simulink model "digital_example_R2017b"  (R2017b)
settings: Solver=VariableStepAuto  StartTime=0.0  StopTime=2  MaxStep=0.001  RelTol=1e-3
undefined symbols (not defined in the file): Kp, T0
settings Model: Creator=Anton Mayorov  LastModifiedBy=bedla

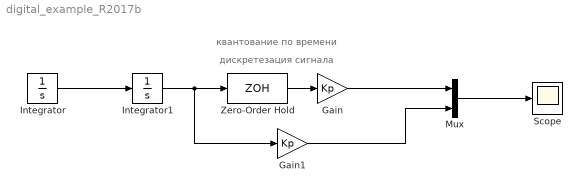
== system digital_example_R2017b ==
  note: дискретезация сигнала
  note: квантование по времени
  Gain : Gain  Gain=Kp
  Gain1 : Gain  Gain=Kp
  Integrator : Integrator  InitialCondition=1
  Integrator1 : Integrator
  Mux : Mux  Inputs=2
  Scope : Scope
  Zero-Order Hold : ZeroOrderHold  SampleTime=T0
  wires:
  Integrator/1 -> Integrator1/1
  Integrator1/1 -> Gain1/1, Zero-Order Hold/1
  Zero-Order Hold/1 -> Gain/1
  Gain/1 -> Mux/1
  Mux/1 -> Scope/1
  Gain1/1 -> Mux/2
